simulink model "blocks"  (R2019a)
settings: Solver=VariableStepAuto  StartTime=0.0  StopTime=10.0  RelTol=1e-3
settings Model: Creator=charles  LastModifiedBy=charles

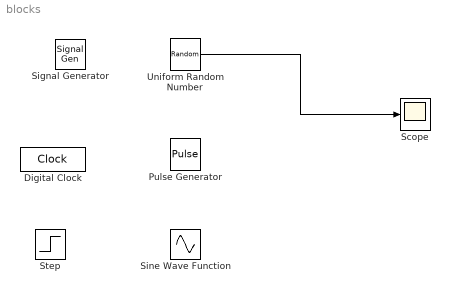
== system blocks ==
  Digital Clock : DigitalClock
  Pulse Generator : DiscretePulseGenerator  PulseType=Time based  Period=10  PulseWidth=5
  Scope : Scope
  Signal Generator : SignalGenerator  Units=rad/sec
  Sine Wave Function : Sin  TimeSource=Use external signal  SampleTime=0
  Step : Step  SampleTime=0
  Uniform Random Number : UniformRandomNumber  Minimum=-2  SampleTime=0.3
  wires:
  Uniform Random Number/1 -> Scope/1
